simulink model "Q1"  (R2018a)
settings: Solver=VariableStepDiscrete  StartTime=0.0  StopTime=0.7  RelTol=1e-3
libraries: powerlib x12
settings Model: Creator=Ataseven  LastModifiedBy=etkiacilan
settings ConfigComp: DVTestSuiteOptimization=CombinedObjectives (Nonlinear Extended)  DVDetectFloatOverflow=off

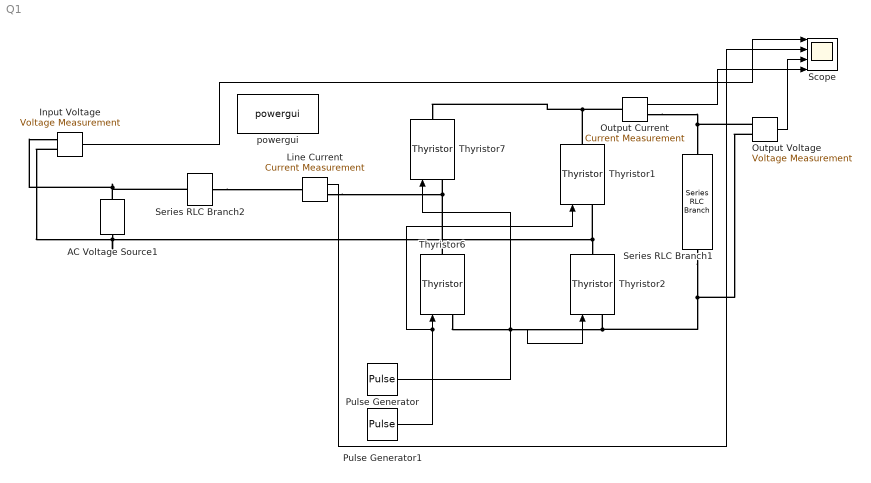
== system Q1 ==
  AC Voltage Source1 : powerlib/Electrical Sources/AC Voltage Source  Amplitude=326.6  Phase=0  Frequency=50  SampleTime=0  Measurements=None  BusType=swing  Pref=10e3  Qref=0  Qmin=-inf  Qmax=+inf
  Input Voltage : powerlib/Measurements/Voltage Measurement  PhasorSimulation=off  OutputType=Complex  PSBequivalent=0
  Line Current : powerlib/Measurements/Current Measurement  PhasorSimulation=off  OutputType=Complex  PSBequivalent=0
  Output Current : powerlib/Measurements/Current Measurement  PhasorSimulation=off  OutputType=Complex  PSBequivalent=0
  Output Voltage : powerlib/Measurements/Voltage Measurement  PhasorSimulation=off  OutputType=Complex  PSBequivalent=0
  Pulse Generator : DiscretePulseGenerator  PulseType=Time based  Amplitude=3  Period=0.02  PulseWidth=5  PhaseDelay=0.02*0.1024
  Pulse Generator1 : DiscretePulseGenerator  PulseType=Time based  Amplitude=3  Period=0.02  PulseWidth=5  PhaseDelay=0.01+0.02*0.1024
  Scope : Scope  NumInputPorts=4
  Series RLC Branch1 : powerlib/Elements/Series RLC Branch  LConnTagsString=__new0  RConnTagsString=__new0  BranchType=RL  Resistance=4  Inductance=200e-3  SetiL0=off  InitialCurrent=0  Capacitance=1e-6  Setx0=off  InitialVoltage=0  Measurements=None
  Series RLC Branch2 : powerlib/Elements/Series RLC Branch  LConnTagsString=__new0  RConnTagsString=__new0  BranchType=L  Resistance=48  Inductance=0.5e-3  SetiL0=off  InitialCurrent=0  Capacitance=1e-6  Setx0=off  InitialVoltage=0  Measurements=None
  Thyristor{1..2,6..7} (4 alike) : powerlib/Power Electronics/Thyristor  Ron=0.001  Lon=0  Vf=0.0001  IC=0  Rs=500  Cs=250e-9  Measurements=off
  powergui : powerlib/powergui  Priority=1  SimulationMode=Discrete  SampleTime=1e-6  frequency=60  Iterations=50  frequencyindice=50  Pbase=100e6  ErrMax=1e-4  UnitsV=kV  UnitsW=MW  buscounter=0  FunctionMessages=off  echomessages=off  EnableUseOfTLC=off  CurrentSourceSwitches=off  DisableSnubberDevices=off  DisableRonSwitches=off  DisableVfSwitches=off  DisplayEquations=off  SolverType=Tustin/Backward Euler (TBE)  Interpol=off  ExternalGateDelay=off  methode=off  Ts=100  x0status=blocks  SPID=on  SwTol=0  HookPort=off  RestoreLinks=warning  ResistiveCurrentMeasurement=off  Frange=[0:2:500]  Ylog=off  Xlog=on  ShowGrid=off  save=off  variable=ZData  structure=ScopeData  ZoomFFT=off  StartTime=0.3  cycles=8  DisplayStyle=1  fundamental=50  FreqAxis=on  MaxFrequency=1000  frequencyindicesteady=1  RmsSteady=1  display=off
  wires:
  Pulse Generator/1 -> Thyristor2/1, Thyristor7/1
  Pulse Generator1/1 -> Thyristor1/1, Thyristor6/1
  Line Current/1 -> Scope/2
  Output Voltage/1 -> Scope/3
  Output Current/1 -> Scope/4
  Input Voltage/1 -> Scope/1
  connections:
  AC Voltage Source1/RConn1 -- Series RLC Branch2/LConn1 -- Input Voltage/LConn1
  AC Voltage Source1/LConn1 -- Thyristor2/RConn1 -- Thyristor1/LConn1 -- Input Voltage/LConn2
  Output Voltage/LConn1 -- Output Current/RConn1 -- Series RLC Branch1/LConn1
  Series RLC Branch1/RConn1 -- Output Voltage/LConn2 -- Thyristor6/LConn1 -- Thyristor2/LConn1
  Thyristor6/RConn1 -- Line Current/RConn1 -- Thyristor7/LConn1
  Output Current/LConn1 -- Thyristor7/RConn1 -- Thyristor1/RConn1
  Series RLC Branch2/RConn1 -- Line Current/LConn1
